simulink model "feedback_forward"  (R2018a)
settings: Solver=VariableStepAuto  StartTime=0.0  StopTime=10.0  RelTol=1e-3
libraries: simulink x2
settings Model: Creator=Dell  LastModifiedBy=Dell

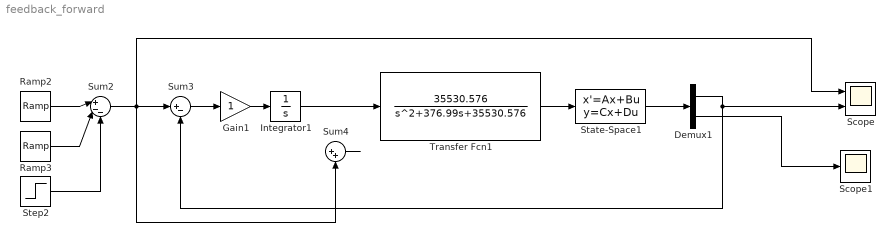
== system feedback_forward ==
  Demux1 : Demux  Outputs=2
  Gain1 : Gain
  Integrator1 : Integrator
  Ramp2 : simulink/Sources/Ramp  slope=150  start=1  InitialOutput=0
  Ramp3 : simulink/Sources/Ramp  slope=150  start=1.1  InitialOutput=0
  Scope : Scope  NumInputPorts=2
  Scope1 : Scope
  State-Space1 : StateSpace  A=-5.443  B=5.063  C=[0.4557;-108.86]  D=[0.5063;101.266]  InitialCondition=0
  Step2 : Step  Time=5  After=15  SampleTime=0
  Sum2 : Sum  Inputs=|+--
  Sum3 : Sum  Inputs=|+-
  Sum4 : Sum  Inputs=|++
  Transfer Fcn1 : TransferFcn  Numerator=[35530.576]  Denominator=[1 376.99 35530.576]
  wires:
  Demux1/1 -> Scope/2, Sum3/2
  Ramp2/1 -> Sum2/1
  Ramp3/1 -> Sum2/2
  Step2/1 -> Sum2/3
  Sum2/1 -> Sum3/1, Scope/1, Sum4/2
  Integrator1/1 -> Transfer Fcn1/1
  State-Space1/1 -> Demux1/1
  Sum3/1 -> Gain1/1
  Transfer Fcn1/1 -> State-Space1/1
  Demux1/2 -> Scope1/1
  Gain1/1 -> Integrator1/1
  Sum4/1 -> ?
